simulink model "OFDM_Rx_HW"  (R2020a)
settings: Solver=FixedStepDiscrete  StartTime=0.0  StopTime=inf  RelTol=1e-3
PostLoadFcn:
  | run ./scripts/filter_setup;
InitFcn:
  | % Set parameters
  | fs = 1e6;
  | 
  | % Load all required variables
  | load('variables/read_addr_data');
  | load('variables/read_addr_cp');
  | load('variables/read_addr_pream');
  | load('variables/read_addr_rx');
  | load('variables/pilot');
  | load('variables/sc_index');
  | load('variables/LTSfreq');
  | load('variables/STSfreq');
  | load('variables/LTSread');
  | load('variables/STSread');
undefined symbols (not defined in the file): CIC_fine_Tx
libraries: dspmlti4 x4, xbsIndex_r4 x1, decimate_rx x1, OFDM_Rx x1, OFDM_Tx x1
settings Model: SimulationMode=accelerator  Creator=njb13206  LastModifiedBy=LDM
settings OptimizationCC: BlockReduction=off  ConditionallyExecuteInputs=off  DefaultParameterBehavior=Inlined
settings DebuggingCC: AlgebraicLoopMsg=error  IntegerOverflowMsg=none  ParameterPrecisionLossMsg=none  IntegerSaturationMsg=none
settings HardwareCC: ProdBitPerPointer=32  ProdBitPerSizeT=32  ProdBitPerPtrDiffT=32  ProdLargestAtomicFloat=None  ProdIntDivRoundTo=Undefined  ProdEndianess=Unspecified  ProdWordSize=32  ProdHWDeviceType=ASIC/FPGA->ASIC/FPGA  TargetBitPerPointer=64  TargetBitPerSizeT=64  TargetBitPerPtrDiffT=64  TargetLongLongMode=on  TargetIntDivRoundTo=Zero  TargetEndianess=LittleEndian  TargetWordSize=64  TargetHWDeviceType=Custom Processor->MATLAB Host Computer  ProdEqTarget=off

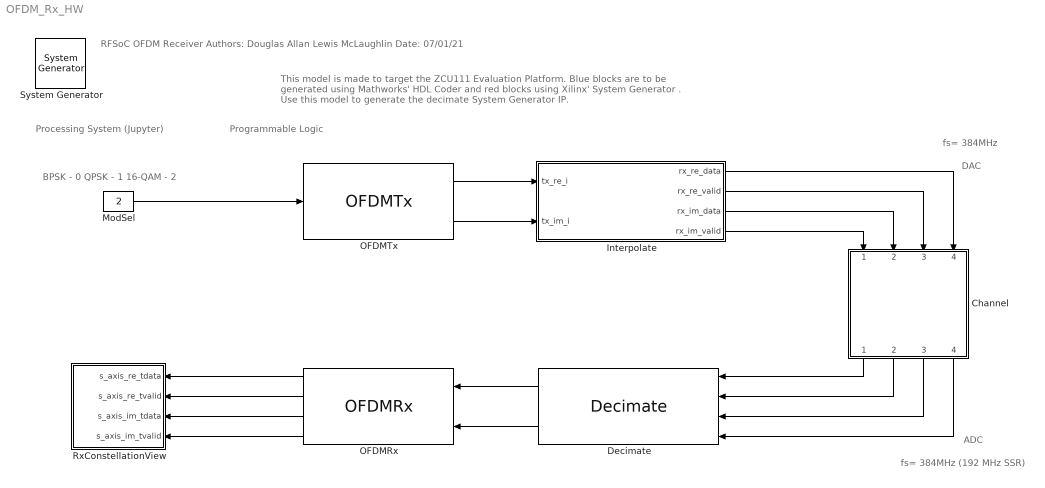
== system OFDM_Rx_HW ==
  note: This model is made to target the ZCU111 Evaluation Platform. Blue blocks are to be generated using Mathworks' HDL Coder and red blocks using Xilinx' System Generator .
      |
      | Use this model to generate the decimate System Generator IP.
  note: Programmable Logic
  note: Processing System (Jupyter)
  note: DAC
  note: BPSK - 0
      | QPSK - 1
      | 16-QAM - 2
  note: fs= 384MHz
  note: ADC
  note: fs= 384MHz (192 MHz SSR)
  note: RFSoC OFDM Receiver
      | Authors: Douglas Allan
      | Lewis McLaughlin
      | Date: 07/01/21
  " System Generator" : xbsIndex_r4/ System Generator  Tag=genX  xilinxfamily=zynquplusRFSOC  part=xczu28dr  speed=-2-e  package=ffvg1517  synthesis_tool=Vivado  clock_wrapper=Clock Enables  directory=C:/Git/rfsoc_ofdm_workspace/models/sys_prj/rx  proj_type=Vivado  Synth_file=Vivado Synthesis Defaults  Impl_file=Vivado Implementation Defaults  testbench=off  simulink_period=1/192e6  sysclk_period=1000/192  dcm_input_clock_period=10  incr_netlist=off  trim_vbits=Everywhere in SubSystem  dbl_ovrd=According to Block Masks  core_generation=According to Block Masks  run_coregen=off  deprecated_control=off  eval_field=0  block_type=sysgen
  "Channel " : Subsystem
  Decimate : decimate_rx/Decimate  SystemSampleTime=-1  Latency=0  AutoFrameSizeCalculation=off
  Interpolate : Subsystem
  ModSel : Constant  Value=2  OutDataTypeStr=fixdt(0,2,0)  SampleTime=1/fs
  OFDMRx : OFDM_Rx/OFDMRx  SystemSampleTime=-1  Latency=0  AutoFrameSizeCalculation=off
  OFDMTx : OFDM_Tx/OFDMTx  SystemSampleTime=-1  Latency=0  AutoFrameSizeCalculation=off
  RxConstellationView : Subsystem
  wires:
  ModSel/1 -> OFDMTx/1
  Interpolate/1(rx_re_data) -> "Channel "/4(chanIn_re)
  OFDMTx/1 -> Interpolate/1(tx_re_i)
  OFDMTx/2 -> Interpolate/2(tx_im_i)
  Interpolate/3(rx_im_data) -> "Channel "/2(chanIn_im)
  Interpolate/2(rx_re_valid) -> "Channel "/3(m_re_tvalid)
  Interpolate/4(rx_im_valid) -> "Channel "/1(m_im_tvalid)
  "Channel "/1(chanOut_re) -> Decimate/1
  "Channel "/3(chanOut_im) -> Decimate/3
  "Channel "/4(tvalid_im_out) -> Decimate/4
  "Channel "/2(tvalid_re_out) -> Decimate/2
  Decimate/1 -> OFDMRx/1
  Decimate/2 -> OFDMRx/2
  OFDMRx/1 -> RxConstellationView/1(s_axis_re_tdata)
  OFDMRx/2 -> RxConstellationView/2(s_axis_re_tvalid)
  OFDMRx/3 -> RxConstellationView/3(s_axis_im_tdata)
  OFDMRx/4 -> RxConstellationView/4(s_axis_im_tvalid)

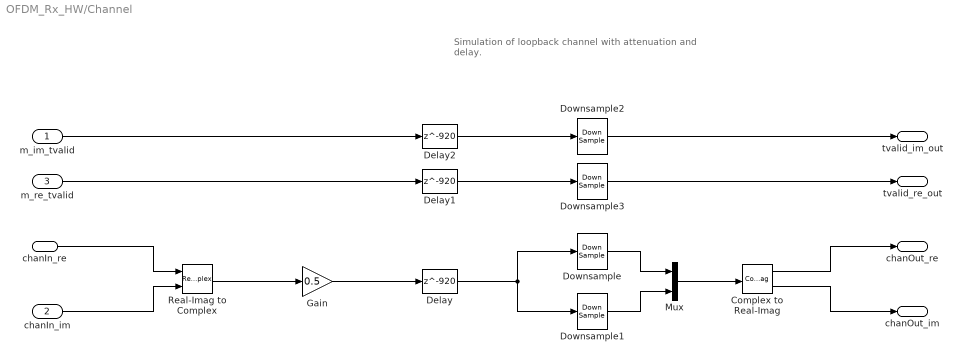
== system OFDM_Rx_HW/Channel  ==
  note: Simulation of loopback channel with attenuation and
      | delay.
  m_im_tvalid : Inport
  chanIn_im : Inport  Port=2
  m_re_tvalid : Inport  Port=3
  chanIn_re : Inport  Port=4
  Complex to Real-Imag : ComplexToRealImag
  Delay : Delay  DelayLength=920
  Delay1 : Delay  DelayLength=920
  Delay2 : Delay  DelayLength=920
  Downsample : DownSample  RateOptions=Allow multirate processing
  Downsample1 : DownSample  phase=1  RateOptions=Allow multirate processing
  Downsample2 : DownSample  RateOptions=Allow multirate processing
  Downsample3 : DownSample  RateOptions=Allow multirate processing
  Gain : Gain  Gain=0.5  ParamDataTypeStr=double  OutDataTypeStr=fixdt(1,16,14)
  Mux : Mux  Inputs=2
  Real-Imag to Complex : RealImagToComplex
  chanOut_re : Outport  VectorParamsAs1DForOutWhenUnconnected=off
  tvalid_re_out : Outport  Port=2  VectorParamsAs1DForOutWhenUnconnected=off
  chanOut_im : Outport  Port=3  VectorParamsAs1DForOutWhenUnconnected=off
  tvalid_im_out : Outport  Port=4  VectorParamsAs1DForOutWhenUnconnected=off
  wires:
  Gain/1 -> Delay/1
  Real-Imag to Complex/1 -> Gain/1
  chanIn_re/1 -> Real-Imag to Complex/1
  chanIn_im/1 -> Real-Imag to Complex/2
  m_re_tvalid/1 -> Delay1/1
  m_im_tvalid/1 -> Delay2/1
  Complex to Real-Imag/1 -> chanOut_re/1
  Complex to Real-Imag/2 -> chanOut_im/1
  Delay1/1 -> Downsample3/1
  Delay2/1 -> Downsample2/1
  Delay/1 -> Downsample1/1, Downsample/1
  Mux/1 -> Complex to Real-Imag/1
  Downsample/1 -> Mux/1
  Downsample1/1 -> Mux/2
  Downsample2/1 -> tvalid_im_out/1
  Downsample3/1 -> tvalid_re_out/1

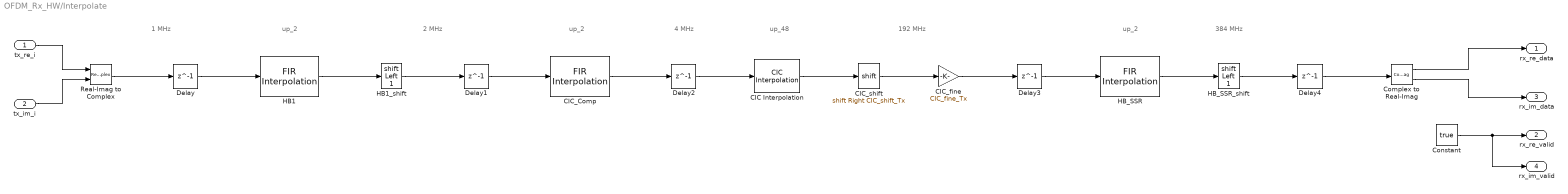
== system OFDM_Rx_HW/Interpolate ==
  note: up_2
  note: 4 MHz
  note: 2 MHz
  note: 1 MHz
  note: 384 MHz
  note: 192 MHz
  note: up_2
  note: up_48
  note: up_2
  tx_re_i : Inport
  tx_im_i : Inport  Port=2
  CIC Interpolation : dspmlti4/CIC Interpolation  filtFrom=Filter object  filtobj=CIC  ftype=Interpolator  R=240  M=1  N=5  filterInternals=Full precision  BPS=[16 16 16 16]  FLPS=0  outputWordLength=32  outputFracLength=0  launchFVT=off  framing=Allow multirate processing  OutputFrames=off
      settings: SourceProductBaseCode=DS
  CIC_Comp : dspmlti4/FIR Interpolation  FilterSource=Dialog parameters  PrivateCoeffs=0  h=WComp.Numerator  L=2  FilterObject=FINTERP  framing=Allow multirate processing  outputBufInitCond=0  roundingMode=Floor  overflowMode=off  firstCoeffMode=Binary point scaling  firstCoeffWordLength=16  firstCoeffFracLength=15  firstCoeffDataTypeStr=fixdt(1,16,15)  firstCoeffMin=[]  firstCoeffMax=[]  firstCoeffLastDataTypeStr=fixdt(1,16,15)  outputMode=Binary point scaling  outputWordLength=16  outputFracLength=14  outputDataTypeStr=fixdt(1,16,14)  outputMin=[]  outputMax=[]  outputLastDataTypeStr=fixdt(1,16,14)
  CIC_fine : Gain  Gain=CIC_fine_Tx  OutDataTypeStr=fixdt(1,16,14)
  CIC_shift : ArithShift  BitShiftNumber=CIC_shift_Tx  BitShiftDirection=Right
  Complex to Real-Imag : ComplexToRealImag
  Constant : Constant  Value=true  SampleTime=1/384e6
  Delay{,1..4} (5 alike) : Delay  DelayLength=1
  HB1 : dspmlti4/FIR Interpolation  FilterSource=Dialog parameters  PrivateCoeffs=0  h=W_HB.Numerator  L=2  FilterObject=FINTERP  framing=Allow multirate processing  outputBufInitCond=0  roundingMode=Floor  overflowMode=off  firstCoeffMode=Binary point scaling  firstCoeffWordLength=16  firstCoeffFracLength=15  firstCoeffDataTypeStr=fixdt(1,16,15)  firstCoeffMin=[]  firstCoeffMax=[]  firstCoeffLastDataTypeStr=fixdt(1,16,15)  outputMode=Binary point scaling  outputWordLength=16  outputFracLength=14  outputDataTypeStr=fixdt(1,16,14)  outputMin=[]  outputMax=[]  outputLastDataTypeStr=fixdt(1,16,14)
  HB1_shift : ArithShift  BitShiftNumber=1  BitShiftDirection=Left
  HB_SSR : dspmlti4/FIR Interpolation  FilterSource=Dialog parameters  PrivateCoeffs=0  h=W_HB_ssr.Numerator  L=2  FilterObject=FINTERP  framing=Allow multirate processing  outputBufInitCond=0  roundingMode=Floor  overflowMode=off  firstCoeffMode=Binary point scaling  firstCoeffWordLength=16  firstCoeffFracLength=15  firstCoeffDataTypeStr=fixdt(1,16,15)  firstCoeffMin=[]  firstCoeffMax=[]  firstCoeffLastDataTypeStr=fixdt(1,16,15)  outputMode=Binary point scaling  outputWordLength=16  outputFracLength=14  outputDataTypeStr=fixdt(1,16,14)  outputMin=[]  outputMax=[]  outputLastDataTypeStr=fixdt(1,16,14)
  HB_SSR_shift : ArithShift  BitShiftNumber=1  BitShiftDirection=Left
  Real-Imag to Complex : RealImagToComplex
  rx_re_data : Outport
  rx_re_valid : Outport  Port=2
  rx_im_data : Outport  Port=3
  rx_im_valid : Outport  Port=4
  wires:
  CIC_fine/1 -> Delay3/1
  CIC_shift/1 -> CIC_fine/1
  HB_SSR_shift/1 -> Delay4/1
  HB_SSR/1 -> HB_SSR_shift/1
  CIC Interpolation/1 -> CIC_shift/1
  HB1_shift/1 -> Delay1/1
  CIC_Comp/1 -> Delay2/1
  HB1/1 -> HB1_shift/1
  Real-Imag to Complex/1 -> Delay/1
  tx_re_i/1 -> Real-Imag to Complex/1
  tx_im_i/1 -> Real-Imag to Complex/2
  Delay/1 -> HB1/1
  Delay1/1 -> CIC_Comp/1
  Delay2/1 -> CIC Interpolation/1
  Delay3/1 -> HB_SSR/1
  Delay4/1 -> Complex to Real-Imag/1
  Complex to Real-Imag/1 -> rx_re_data/1
  Complex to Real-Imag/2 -> rx_im_data/1
  Constant/1 -> rx_im_valid/1, rx_re_valid/1

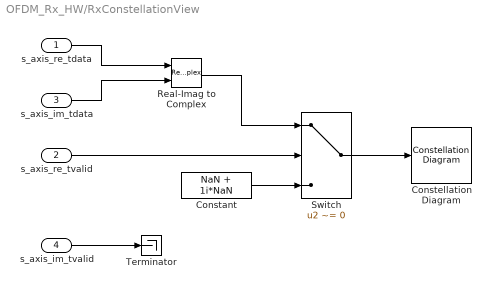
== system OFDM_Rx_HW/RxConstellationView ==
  s_axis_re_tdata : Inport
  s_axis_re_tvalid : Inport  Port=2
  s_axis_im_tdata : Inport  Port=3
  s_axis_im_tvalid : Inport  Port=4
  Constant : Constant  Value=NaN + 1i*NaN  OutDataTypeStr=double  SampleTime=-1
  Constellation Diagram : ConstellationDiagram
  Real-Imag to Complex : RealImagToComplex
  Switch : Switch  Criteria=u2 ~= 0
  Terminator : Terminator
  wires:
  Switch/1 -> Constellation Diagram/1
  Constant/1 -> Switch/3
  s_axis_re_tvalid/1 -> Switch/2
  Real-Imag to Complex/1 -> Switch/1
  s_axis_im_tvalid/1 -> Terminator/1
  s_axis_re_tdata/1 -> Real-Imag to Complex/1
  s_axis_im_tdata/1 -> Real-Imag to Complex/2
